simulink model "Two_Link_Newton_Euler"  (R2021b)
settings: Solver=FixedStepAuto  StartTime=0.0  StopTime=10.0  FixedStep=0.001  RelTol=1e-3
undefined symbols (not defined in the file): g, I1, I2, L1, L2, Lac, Loc, M1, M2, Mp
settings Model: Creator=salva  LastModifiedBy=salva
settings OptimizationCC: DefaultParameterBehavior=Inlined  EnhancedBackFolding=on  PassReuseOutputArgsAs=Individual arguments  ZeroExternalMemoryAtStartup=off  ZeroInternalMemoryAtStartup=off  OptimizeBlockOrder=speed  DifferentSizesBufferReuse=on  OptimizationCustomize=off  EfficientTunableParamExpr=on
settings DebuggingCC: ParameterTunabilityLossMsg=error
settings SFSimCC: MATLABDynamicMemAlloc=off
settings RTWCC: Description=Embedded Coder  SystemTargetFile=ert.tlc  TemplateMakefile=ert_default_tmf
settings CodeAppCC: ForceParamTrailComments=on  IgnoreCustomStorageClasses=off  OperatorAnnotations=on  SimulinkDataObjDesc=on  SFDataObjDesc=on  InsertBlockDesc=on
settings ERTTargetCC: TargetLangStandard=C99 (ISO)  GenerateSampleERTMain=on  InlinedParameterPlacement=NonHierarchical  ERTCustomFileTemplate=example_file_process.tlc

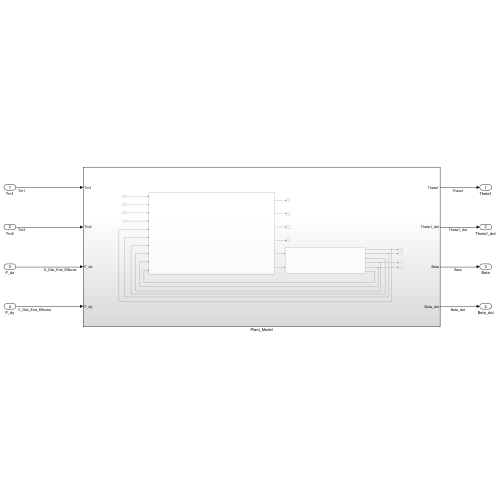
[thumbnail: Simulink's stored preview of the top-level diagram]
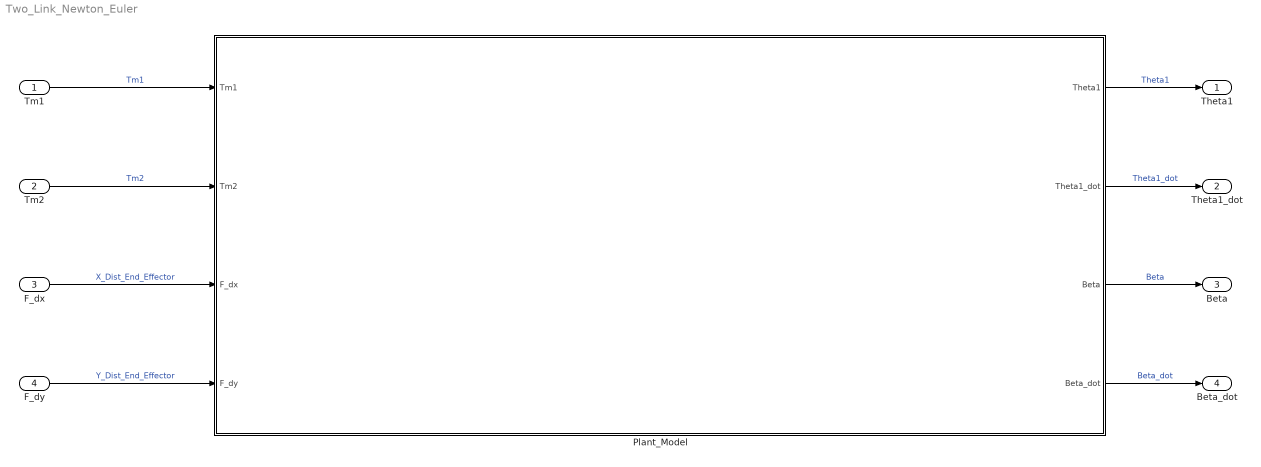
== system Two_Link_Newton_Euler ==
  Tm1 : Inport
  Tm2 : Inport  Port=2
  F_dx : Inport  Port=3
  F_dy : Inport  Port=4
  Plant_Model : Subsystem
  Theta1 : Outport
  Theta1_dot : Outport  Port=2
  Beta : Outport  Port=3
  Beta_dot : Outport  Port=4
  wires:
  F_dy/1 -> Plant_Model/4(F_dy)  "Y_Dist_End_Effector"
  Tm2/1 -> Plant_Model/2(Tm2)  "Tm2"
  Tm1/1 -> Plant_Model/1(Tm1)  "Tm1"
  F_dx/1 -> Plant_Model/3(F_dx)  "X_Dist_End_Effector"
  Plant_Model/2(Theta1_dot) -> Theta1_dot/1  "Theta1_dot"
  Plant_Model/3(Beta) -> Beta/1  "Beta"
  Plant_Model/4(Beta_dot) -> Beta_dot/1  "Beta_dot"
  Plant_Model/1(Theta1) -> Theta1/1  "Theta1"

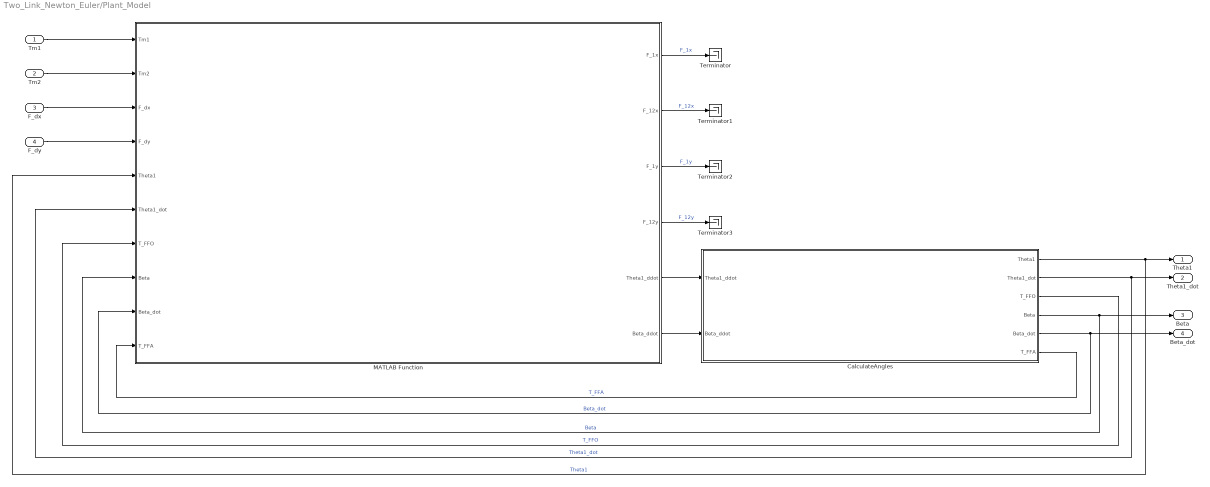
== system Two_Link_Newton_Euler/Plant_Model ==
  Tm1 : Inport
  Tm2 : Inport  Port=2
  F_dx : Inport  Port=3
  F_dy : Inport  Port=4
  CalculateAngles : Subsystem
  MATLAB Function : MATLAB Function  TreatAsAtomicUnit=on
  Terminator{,1..3} (4 alike) : Terminator
  Theta1 : Outport
  Theta1_dot : Outport  Port=2
  Beta : Outport  Port=3
  Beta_dot : Outport  Port=4
  wires:
  MATLAB Function/2(F_12x) -> Terminator1/1  "F_12x"
  CalculateAngles/1(Theta1) -> Theta1/1, MATLAB Function/5(Theta1)  "Theta1"
  F_dx/1 -> MATLAB Function/3(F_dx)
  CalculateAngles/5(Beta_dot) -> MATLAB Function/9(Beta_dot), Beta_dot/1  "Beta_dot"
  CalculateAngles/2(Theta1_dot) -> Theta1_dot/1, MATLAB Function/6(Theta1_dot)  "Theta1_dot"
  MATLAB Function/5(Theta1_ddot) -> CalculateAngles/1(Theta1_ddot)
  CalculateAngles/4(Beta) -> Beta/1, MATLAB Function/8(Beta)  "Beta"
  CalculateAngles/3(T_FFO) -> MATLAB Function/7(T_FFO)  "T_FFO"
  CalculateAngles/6(T_FFA) -> MATLAB Function/10(T_FFA)  "T_FFA"
  MATLAB Function/1(F_1x) -> Terminator/1  "F_1x"
  MATLAB Function/4(F_12y) -> Terminator3/1  "F_12y"
  MATLAB Function/3(F_1y) -> Terminator2/1  "F_1y"
  Tm2/1 -> MATLAB Function/2(Tm2)
  Tm1/1 -> MATLAB Function/1(Tm1)
  F_dy/1 -> MATLAB Function/4(F_dy)
  MATLAB Function/6(Beta_ddot) -> CalculateAngles/2(Beta_ddot)

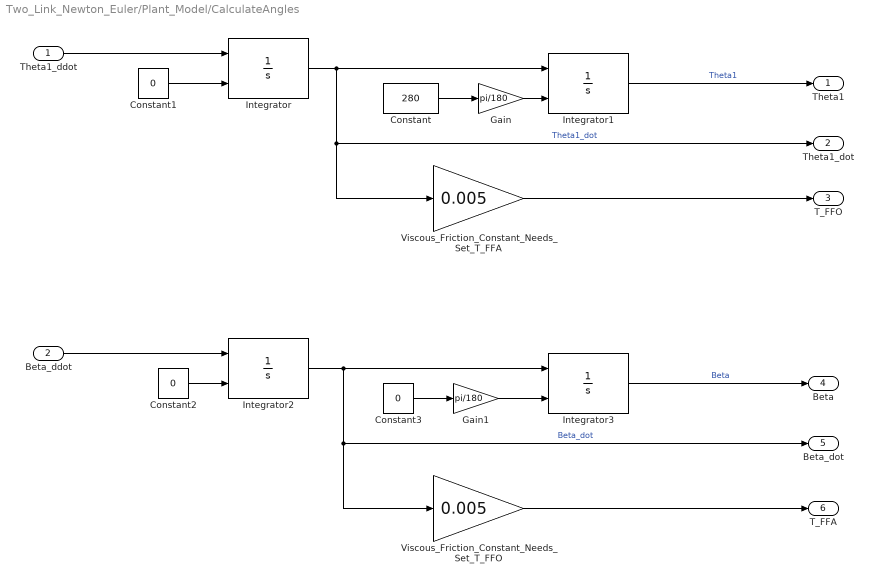
== system Two_Link_Newton_Euler/Plant_Model/CalculateAngles ==
  Theta1_ddot : Inport
  Beta_ddot : Inport  Port=2
  Constant : Constant  Value=280
  Constant1 : Constant  Value=0
  Constant2 : Constant  Value=0
  Constant3 : Constant  Value=0
  Gain : Gain  Gain=pi/180
  Gain1 : Gain  Gain=pi/180
  Integrator{,1..3} (4 alike) : Integrator  InitialConditionSource=external
  Viscous_Friction_Constant_Needs_Set_T_FFA : Gain  Gain=0.005
  Viscous_Friction_Constant_Needs_Set_T_FFO : Gain  Gain=0.005
  Theta1 : Outport
  Theta1_dot : Outport  Port=2
  T_FFO : Outport  Port=3
  Beta : Outport  Port=4
  Beta_dot : Outport  Port=5
  T_FFA : Outport  Port=6
  wires:
  Integrator2/1 -> Integrator3/1, Beta_dot/1, Viscous_Friction_Constant_Needs_Set_T_FFO/1  "Beta_dot"
  Integrator3/1 -> Beta/1  "Beta"
  Theta1_ddot/1 -> Integrator/1
  Viscous_Friction_Constant_Needs_Set_T_FFA/1 -> T_FFO/1
  Viscous_Friction_Constant_Needs_Set_T_FFO/1 -> T_FFA/1
  Beta_ddot/1 -> Integrator2/1
  Integrator1/1 -> Theta1/1  "Theta1"
  Integrator/1 -> Theta1_dot/1, Viscous_Friction_Constant_Needs_Set_T_FFA/1, Integrator1/1  "Theta1_dot"
  Constant/1 -> Gain/1
  Gain/1 -> Integrator1/2
  Constant1/1 -> Integrator/2
  Constant2/1 -> Integrator2/2
  Constant3/1 -> Gain1/1
  Gain1/1 -> Integrator3/2

== matlab function Two_Link_Newton_Euler/Plant_Model/MATLAB Function ==
  data: Tm1 input; F_1x output; Tm2 input; F_dx input; F_dy input; Theta1 input; Theta1_dot input; T_FFO input; Beta input; Beta_dot input; T_FFA input; F_12x output; F_1y output; F_12y output; Theta1_ddot output; Beta_ddot output; M1 parameter; M2 parameter; L1 parameter; L2 parameter; I1 parameter; I2 parameter; Lac parameter; Loc parameter; Mp parameter; g parameter
function [F_1x,F_12x,F_1y,F_12y, Theta1_ddot,Beta_ddot] =Two_Link_F_Kinetics(Tm1,Tm2,F_dx,F_dy,Theta1,Theta1_dot,T_FFO,Beta, Beta_dot,T_FFA, M1, M2, L1, L2, I1, I2, Lac, Loc, Mp, g)
%% Calculation Simplifications
S1 = sin(Theta1);
C1 = cos(Theta1);
Theta2 = Theta1+Beta;
S2 = sin(Theta2);
C2 = cos(Theta2);
S3 = sin(Beta);
C3 = cos(Beta);
Theta1_dot_sq = Theta1_dot*Theta1_dot;
Theta2_dot_sq = (Theta1_dot+Beta_dot)*(Theta1_dot+Beta_dot);
%% Setting Up the Forward Newton Euler Matrix
A = zeros(6,6); % Define a Zero matrix of 6x6 size
B = zeros(6,1); % Define a Zero Vector
% Indexing Row 1 Of A which is Equation 1.
% -F_1x + F_12x + (M1*Loc*sin(Theta1))*Theta1_ddot 
% Cleaned up Equation
% F_1x + F_12x + (M1*Loc*S1)*Theta1_ddot
A(1,1) = -1; 
A(1,2) = 1;
A(1,3) = 0;
A(1,4) = 0;
A(1,5) = (M1*Loc*S1);
A(1,6) = 0;

% Indexing Row 2 Of A which is Equation 2.
% -F_1y + F_12y -(M1*Loc*cos(Theta1))*Theta1_ddot 
% Cleaned up Equation
% -F_1y + F_12y -(M1*Loc*C1)*Theta1_ddot 
A(2,1) = 0; 
A(2,2) = 0;
A(2,3) = -1;
A(2,4) = 1;
A(2,5) = -(M1*Loc*C1);
A(2,6) = 0;

% Indexing Row 3 Of A which is Equation 3.
% - L1*sin(Theta1)*F_12x + L1*cos(Theta1)*F_12y - (I1+(M1*(Loc^2)))*Theta1_ddot
% Cleaned up Equation
% -(L1*S1)*F_12x +(L1*C1)*F_12y -(I1+(M1*(Loc*Loc)))*Theta1_ddot
A(3,1) = 0; 
A(3,2) = -(L1*S1);
A(3,3) = 0;
A(3,4) = (L1*C1);
A(3,5) = -(I1+(M1*(Loc*Loc)));
A(3,6) = 0;

% Indexing Row 4 Of A which is Equation 4.
% -F_12x + M2*((L1*sin(Theta1))+(Lac*sin(Beta+Theta1)))*Theta1_ddot +
% (M2*Lac*sin(Beta+Theta1))*Beta_ddot
% Cleaned up Equation
% -F_12x + M2*((L1*S1)+(Lac*S2))*Theta1_ddot + (M2*Lac*S2)*Beta_ddot
A(4,1) = 0; 
A(4,2) = -1;
A(4,3) = 0;
A(4,4) = 0;
A(4,5) = M2*((L1*S1)+(Lac*S2));
A(4,6) = (M2*Lac*S2);

% Indexing Row 5 Of A which is Equation 5.
% -F_12y - M2*((L1*cos(Theta1))+(Lac*cos(Beta+Theta1)))*Theta1_ddot -
% (M2*Lac*cos(Beta+Theta1))*Beta_ddot
% Cleaned up Equation
% -F_12y - M2*((L1*C1)+(Lac*C2))*Theta1_ddot -(M2*Lac*C2)*Beta_ddot
A(5,1) = 0; 
A(5,2) = 0;
A(5,3) = 0;
A(5,4) = -1;
A(5,5) = - M2*((L1*C1)+(Lac*C2));
A(5,6) = -(M2*Lac*C2);

% Indexing Row 6 Of A which is Equation 6.
% (I2+((M2*Lac)*(L1*cos(Beta)+Lac)))*Theta1_ddot + ((M2*Lac^2)+I2)*Beta_ddot
% Cleaned Up Equation
% (I2+((M2*Lac)*(L1*C3+Lac)))*Theta1_ddot + ((M2*Lac*Lac)+I2)*Beta_ddot
A(6,1) = 0; 
A(6,2) = 0;
A(6,3) = 0;
A(6,4) = 0;
A(6,5) = (I2+((M2*Lac)*(L1*C3+Lac)));
A(6,6) = ((M2*Lac*Lac)+I2);

% Setting Up the B Matrix

% Indexing Row 1 of B which is RHS of EQ1
% -(M1*Loc*cos(Theta1)*(Theta1_dot^2))
% Cleaned Up Equation
% -(M1*Loc*C1*(Theta1_dot*Theta1_dot))
% -(M1*Loc*C1*Theta1_dot_sq)
B(1) = -(M1*Loc*C1*Theta1_dot_sq);

% Indexing Row 2 of B which is RHS of EQ2
% -(M1*Loc*sin(Theta1)*(Theta1_dot^2))+(M1*g)
% Cleaned Up Equation
% -(M1*Loc*S1*(Theta1_dot*Theta1_dot))+(M1*g)
% -(M1*Loc*S1*(Theta1_dot_sq))+(M1*g)
B(2) = -(M1*Loc*S1*(Theta1_dot_sq))+(M1*g);

% Indexing Row 3 of B which is RHS of EQ3
% -Tm1+T_FFO-T_FFA+(Loc*M1*g*cos(Theta1))-Tm2
% Cleaned Up Equation
% -Tm1+T_FFO-T_FFA+(Loc*M1*g*C1)-Tm2
B(3) = -Tm1+T_FFO-T_FFA+(Loc*M1*g*C1)-Tm2;

% Indexing Row 4 of B which is RHS of EQ4
% - (M2*L1*cos(Theta1)*(Theta1_dot^2)) - M2*Lac*cos(Beta+Theta1)*(Beta_dot+Theta1_dot)^2 - F_dx
% Cleaned Up Equation
% -(M2*L1*C1*(Theta1_dot*Theta1_dot)) - (M2* Lac*C2*(Beta_dot+Theta1_dot)*(Beta_dot+Theta1_dot)) - F_dx
% -(M2*L1*C1*(Theta1_dot_sq)) - (M2*Lac*C2*Theta2_dot_sq) - F_dx
B(4) = -(M2*L1*C1*(Theta1_dot_sq)) - (M2*Lac*C2*Theta2_dot_sq) - F_dx;

% Indexing Row 5 of B which is RHS of EQ5
% -(M2*L1*sin(Theta1)*(Theta1_dot^2)) - M2*Lac*sin(Beta+Theta1)*(Beta_dot+Theta1_dot)^2 + g*(M2+Mp) + F_dy
% Cleaned Up Equation
% -(M2*L1*S1*(Theta1_dot*Theta1_dot)) - (M2*Lac*S2*(Beta_dot+Theta1_dot)*(Beta_dot+Theta1_dot)) + g*(M2+Mp) + F_dy
% -(M2*L1*S1*(Theta1_dot_sq)) - (M2*Lac*S2*Theta2_dot_sq) + g*(M2+Mp) + F_dy
B(5) = -(M2*L1*S1*(Theta1_dot_sq)) - (M2*Lac*S2*Theta2_dot_sq) + g*(M2+Mp) + F_dy;

% Indexing Row 6 of B which is RHS of EQ6
% Tm2 - T_FFA - cos(Beta+Theta1)*((Lac*M2*g)+(L2*(Mp*g+F_dy))-(L2*sin(Beta+Theta1)*F_dx)-(M2*Lac*L1*sin(Beta)*(Theta1_dot^2))
% Cleaned Up Equation
% Tm2 - T_FFA - C2*((Lac*M2*g)+(L2*(Mp*g+F_dy)))-(L2*S2*F_dx) -(M2*Lac*L1*S3*(Theta1_dot*Theta1_dot))
% Tm2 - T_FFA - C2*((Lac*M2*g)+(L2*(Mp*g+F_dy)))-(L2*S2*F_dx) -(M2*Lac*L1*S3*(Theta1_dot_sq))
B(6) = Tm2 - T_FFA - C2*((Lac*M2*g)+(L2*(Mp*g+F_dy)))-(L2*S2*F_dx) -(M2*Lac*L1*S3*(Theta1_dot_sq));


Y = A\B;

F_1x = Y(1);
F_12x = Y(2);
F_1y = Y(3);
F_12y = Y(4);
Theta1_ddot = Y(5);
Beta_ddot = Y(6);
